simulink model "Simple_noL"  (R2020a)
settings: Solver=ode23  StartTime=0.0  StopTime=10.0  MaxStep=1e-2  RelTol=1e-3
libraries: simulink x4, fmu_me_lib x4
settings Model: Creator=Bob  LastModifiedBy=meagh
settings SFSimCC: CustomCodeUndefinedFunction=UseInterfaceOnly

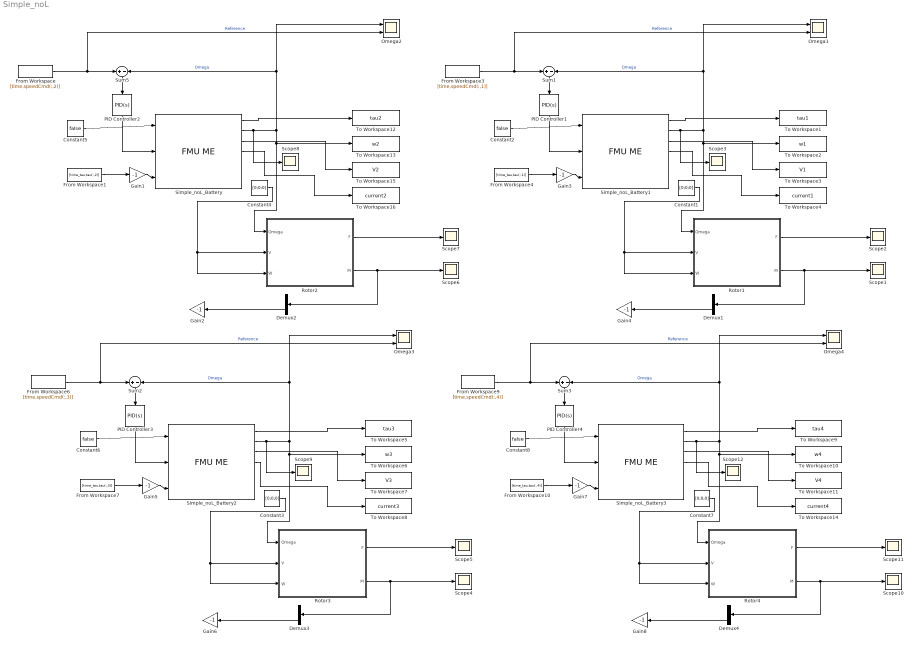
== system Simple_noL ==
  Constant{1,3..4,7} (4 alike) : Constant  Value=[0;0;0]
  Constant{2,5..6,8} (4 alike) : Constant  Value=false  OutDataTypeStr=boolean
  Demux{1..4} (4 alike) : Demux  Outputs=3
  From Workspace : FromWorkspace  VariableName=[time,speedCmd(:,2)]
  From Workspace1 : FromWorkspace  VariableName=[time_tau,tau(:,2)]
  From Workspace10 : FromWorkspace  VariableName=[time_tau,tau(:,4)]
  From Workspace3 : FromWorkspace  VariableName=[time,speedCmd(:,1)]
  From Workspace4 : FromWorkspace  VariableName=[time_tau,tau(:,1)]
  From Workspace6 : FromWorkspace  VariableName=[time,speedCmd(:,3)]
  From Workspace7 : FromWorkspace  VariableName=[time_tau,tau(:,3)]
  From Workspace9 : FromWorkspace  VariableName=[time,speedCmd(:,4)]
  Gain{1..8} (8 alike) : Gain  Gain=-1
  Omega{1..4} (4 alike) : Scope  NumInputPorts=2
  PID Controller{1..4} (4 alike) : simulink/Continuous/PID Controller  Controller=PID  Form=Parallel  TimeDomain=Continuous-time  UseExternalTs=off  SampleTime=-1  IntegratorMethod=Forward Euler  FilterMethod=Forward Euler  ControllerParametersSource=internal  P=0.0184*0.2  I=0.0184  D=0  UseFilter=on  N=100  TunerSelectOption=Transfer Function Based (PID Tuner App)  InitialConditionSource=internal  InitialConditionForIntegrator=0  InitialConditionForFilter=0  DifferentiatorICPrevScaledInput=0  ExternalReset=none  TrackingMode=off  Kt=1  LimitOutput=off  UpperSaturationLimit=inf  LowerSaturationLimit=-inf  LinearizeAsGain=on  AntiWindupMode=none  Kb=1  POutMin=[]  POutMax=[]  IOutMin=[]  IOutMax=[]  DOutMin=[]  DOutMax=[]  NOutMin=[]  NOutMax=[]  SumOutMin=[]  SumOutMax=[]  SaturationOutMin=[]  SaturationOutMax=[]  PParamMin=[]  PParamMax=[]  IParamMin=[]  IParamMax=[]  DParamMin=[]  DParamMax=[]  NParamMin=[]  NParamMax=[]  KbParamMin=[]  KbParamMax=[]  KtParamMin=[]  KtParamMax=[]  KbOutMin=[]  KbOutMax=[]  KtOutMin=[]  KtOutMax=[]  IntegratorOutMin=[]  IntegratorOutMax=[]  FilterOutMin=[]  FilterOutMax=[]  SumI1OutMin=[]  SumI1OutMax=[]  SumI2OutMin=[]  SumI2OutMax=[]  SumI3OutMin=[]  SumI3OutMax=[]  SumI4OutMin=[]  SumI4OutMax=[]  SumDOutMin=[]  SumDOutMax=[]  DifferentiatorOutMin=[]  DifferentiatorOutMax=[]  FilterDiffOutCoefMin=[]  FilterDiffOutCoefMax=[]  ReciprocalOutMin=[]  ReciprocalOutMax=[]  SumDenOutMin=[]  SumDenOutMax=[]  SumNumOutMin=[]  SumNumOutMax=[]  DivideOutMin=[]  DivideOutMax=[]  UdiffTsProdOutMin=[]  UdiffTsProdOutMax=[]  NTsProdOutMin=[]  NTsProdOutMax=[]  UintegralTsProdOutMin=[]  UintegralTsProdOutMax=[]  UngainTsProdOutMin=[]  UngainTsProdOutMax=[]  IntegratorContinuousStateAttributes=''  IntegratorStateMustResolveToSignalObject=off  IntegratorRTWStateStorageClass=Auto  FilterContinuousStateAttributes=''  FilterStateMustResolveToSignalObject=off  FilterRTWStateStorageClass=Auto  ParallelPVariant=InternalParameters  IdealPVariant=Disabled  IVariant=InternalParameters  DVariant=InternalParameters  IntegratorVariant=Continuous  SatVariant=Disabled  AWVariant=Passthrough  PCopyVariant=Disabled  TRVariant=Disabled  FdbkBlocksVariant=Forward  IdealPFdbkVariant=Disabled  SatFdbkVariant=Disabled  DerivativeFilterVariant=ContFilter  NVariant=InternalParameters  NCopyVariant=Disabled  FilterICVariant=InternalICsFilter  IntegratorICVariant=InternalICs  ExternalResetVariant=Disabled  TRSumVariant=Passthrough  SumFdbkVariant=Disabled  SumVariant=Sum_PID  TsampFilterVariant=InternalTs  TsampNgainVariant=Passthrough  TsampIntegralVariant=Passthrough
  Rotor1 : Subsystem
  Rotor2 : Subsystem
  Rotor3 : Subsystem
  Rotor4 : Subsystem
  Scope{1..12} (12 alike) : Scope
  Simple_noL_Battery{,1..3} (4 alike) : fmu_me_lib/FMU ME  Description=Simulates an FMU for Model Exchange 1.0 or Model Exchange 2.0.  dummy=0
  Sum{1..3,5} (4 alike) : Sum  Inputs=+|-
  To Workspace1 : ToWorkspace  VariableName=tau1  SaveFormat=Timeseries  SampleTime=-1
  To Workspace10 : ToWorkspace  VariableName=w4  SaveFormat=Timeseries  SampleTime=-1
  To Workspace11 : ToWorkspace  VariableName=V4  SaveFormat=Timeseries  SampleTime=-1
  To Workspace12 : ToWorkspace  VariableName=tau2  SaveFormat=Timeseries  SampleTime=-1
  To Workspace13 : ToWorkspace  VariableName=w2  SaveFormat=Timeseries  SampleTime=-1
  To Workspace14 : ToWorkspace  VariableName=current4  SaveFormat=Timeseries  SampleTime=-1
  To Workspace15 : ToWorkspace  VariableName=V2  SaveFormat=Timeseries  SampleTime=-1
  To Workspace16 : ToWorkspace  VariableName=current2  SaveFormat=Timeseries  SampleTime=-1
  To Workspace2 : ToWorkspace  VariableName=w1  SaveFormat=Timeseries  SampleTime=-1
  To Workspace3 : ToWorkspace  VariableName=V1  SaveFormat=Timeseries  SampleTime=-1
  To Workspace4 : ToWorkspace  VariableName=current1  SaveFormat=Timeseries  SampleTime=-1
  To Workspace5 : ToWorkspace  VariableName=tau3  SaveFormat=Timeseries  SampleTime=-1
  To Workspace6 : ToWorkspace  VariableName=w3  SaveFormat=Timeseries  SampleTime=-1
  To Workspace7 : ToWorkspace  VariableName=V3  SaveFormat=Timeseries  SampleTime=-1
  To Workspace8 : ToWorkspace  VariableName=current3  SaveFormat=Timeseries  SampleTime=-1
  To Workspace9 : ToWorkspace  VariableName=tau4  SaveFormat=Timeseries  SampleTime=-1
  wires:
  Constant5/1 -> Simple_noL_Battery/1
  Rotor2/1(F) -> Scope7/1
  Simple_noL_Battery/1 -> To Workspace12/1
  Simple_noL_Battery/4 -> To Workspace16/1
  Simple_noL_Battery/3 -> To Workspace15/1
  Simple_noL_Battery/2 -> Scope8/1, To Workspace13/1, Rotor2/1(Omega), Omega2/1, Sum5/2  "Omega"
  Rotor2/2(M) -> Demux2/1, Scope6/1
  Constant4/1 -> Rotor2/3(W), Rotor2/2(V)
  From Workspace/1 -> Omega2/2, Sum5/1  "Reference"
  Demux2/3 -> Gain2/1
  PID Controller2/1 -> Simple_noL_Battery/2
  Sum5/1 -> PID Controller2/1
  From Workspace1/1 -> Gain1/1
  Gain1/1 -> Simple_noL_Battery/3
  From Workspace3/1 -> Omega1/2, Sum1/1  "Reference"
  Gain3/1 -> Simple_noL_Battery1/3
  Simple_noL_Battery1/2 -> Scope3/1, To Workspace2/1, Rotor1/1(Omega), Omega1/1, Sum1/2  "Omega"
  Simple_noL_Battery1/3 -> To Workspace3/1
  PID Controller1/1 -> Simple_noL_Battery1/2
  Simple_noL_Battery1/1 -> To Workspace1/1
  Constant1/1 -> Rotor1/3(W), Rotor1/2(V)
  Rotor1/1(F) -> Scope2/1
  Demux1/3 -> Gain4/1
  Sum1/1 -> PID Controller1/1
  Constant2/1 -> Simple_noL_Battery1/1
  Rotor1/2(M) -> Demux1/1, Scope1/1
  Simple_noL_Battery1/4 -> To Workspace4/1
  From Workspace4/1 -> Gain3/1
  PID Controller3/1 -> Simple_noL_Battery2/2
  Simple_noL_Battery2/2 -> Scope9/1, To Workspace6/1, Rotor3/1(Omega), Omega3/1, Sum2/2  "Omega"
  Gain5/1 -> Simple_noL_Battery2/3
  From Workspace6/1 -> Omega3/2, Sum2/1  "Reference"
  From Workspace7/1 -> Gain5/1
  Simple_noL_Battery2/4 -> To Workspace8/1
  Sum2/1 -> PID Controller3/1
  Demux3/3 -> Gain6/1
  Constant3/1 -> Rotor3/3(W), Rotor3/2(V)
  Simple_noL_Battery2/3 -> To Workspace7/1
  Simple_noL_Battery2/1 -> To Workspace5/1
  Rotor3/2(M) -> Demux3/1, Scope4/1
  Rotor3/1(F) -> Scope5/1
  Constant6/1 -> Simple_noL_Battery2/1
  PID Controller4/1 -> Simple_noL_Battery3/2
  Simple_noL_Battery3/2 -> Scope12/1, To Workspace10/1, Rotor4/1(Omega), Omega4/1, Sum3/2  "Omega"
  Gain7/1 -> Simple_noL_Battery3/3
  From Workspace9/1 -> Omega4/2, Sum3/1  "Reference"
  From Workspace10/1 -> Gain7/1
  Simple_noL_Battery3/4 -> To Workspace14/1
  Sum3/1 -> PID Controller4/1
  Demux4/3 -> Gain8/1
  Constant7/1 -> Rotor4/3(W), Rotor4/2(V)
  Simple_noL_Battery3/3 -> To Workspace11/1
  Simple_noL_Battery3/1 -> To Workspace9/1
  Rotor4/2(M) -> Demux4/1, Scope10/1
  Rotor4/1(F) -> Scope11/1
  Constant8/1 -> Simple_noL_Battery3/1

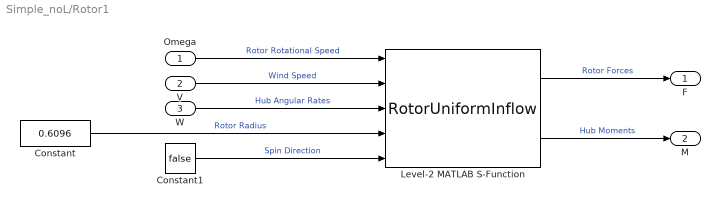
== system Simple_noL/Rotor1 ==
  Omega : Inport  OutDataTypeStr=double
  V : Inport  Port=2  OutDataTypeStr=double
  W : Inport  Port=3  OutDataTypeStr=double
  Constant : Constant  Value=0.6096
  Constant1 : Constant  Value=false  OutDataTypeStr=boolean
  Level-2 MATLAB S-Function : M-S-Function  FunctionName=RotorUniformInflow
  F : Outport  OutDataTypeStr=double  VectorParamsAs1DForOutWhenUnconnected=off
  M : Outport  Port=2  OutDataTypeStr=double  VectorParamsAs1DForOutWhenUnconnected=off
  wires:
  Level-2 MATLAB S-Function/2 -> M/1  "Hub Moments"
  Constant/1 -> Level-2 MATLAB S-Function/4  "Rotor Radius"
  Constant1/1 -> Level-2 MATLAB S-Function/5  "Spin Direction"
  Omega/1 -> Level-2 MATLAB S-Function/1  "Rotor Rotational Speed"
  V/1 -> Level-2 MATLAB S-Function/2  "Wind Speed"
  Level-2 MATLAB S-Function/1 -> F/1  "Rotor Forces"
  W/1 -> Level-2 MATLAB S-Function/3  "Hub Angular Rates"

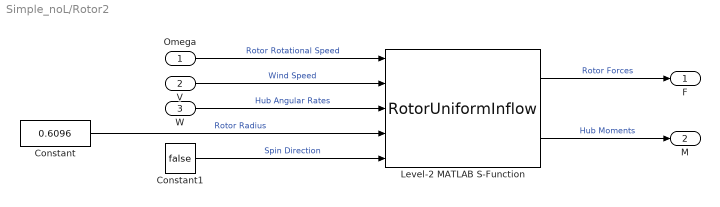
== system Simple_noL/Rotor2 ==
  Omega : Inport  OutDataTypeStr=double
  V : Inport  Port=2  OutDataTypeStr=double
  W : Inport  Port=3  OutDataTypeStr=double
  Constant : Constant  Value=0.6096
  Constant1 : Constant  Value=false  OutDataTypeStr=boolean
  Level-2 MATLAB S-Function : M-S-Function  FunctionName=RotorUniformInflow
  F : Outport  OutDataTypeStr=double  VectorParamsAs1DForOutWhenUnconnected=off
  M : Outport  Port=2  OutDataTypeStr=double  VectorParamsAs1DForOutWhenUnconnected=off
  wires:
  Level-2 MATLAB S-Function/2 -> M/1  "Hub Moments"
  Constant/1 -> Level-2 MATLAB S-Function/4  "Rotor Radius"
  Constant1/1 -> Level-2 MATLAB S-Function/5  "Spin Direction"
  Omega/1 -> Level-2 MATLAB S-Function/1  "Rotor Rotational Speed"
  V/1 -> Level-2 MATLAB S-Function/2  "Wind Speed"
  Level-2 MATLAB S-Function/1 -> F/1  "Rotor Forces"
  W/1 -> Level-2 MATLAB S-Function/3  "Hub Angular Rates"

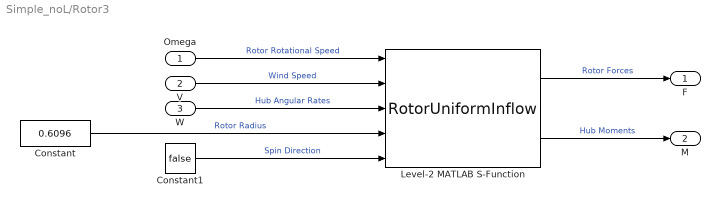
== system Simple_noL/Rotor3 ==
  Omega : Inport  OutDataTypeStr=double
  V : Inport  Port=2  OutDataTypeStr=double
  W : Inport  Port=3  OutDataTypeStr=double
  Constant : Constant  Value=0.6096
  Constant1 : Constant  Value=false  OutDataTypeStr=boolean
  Level-2 MATLAB S-Function : M-S-Function  FunctionName=RotorUniformInflow
  F : Outport  OutDataTypeStr=double  VectorParamsAs1DForOutWhenUnconnected=off
  M : Outport  Port=2  OutDataTypeStr=double  VectorParamsAs1DForOutWhenUnconnected=off
  wires:
  Level-2 MATLAB S-Function/2 -> M/1  "Hub Moments"
  Constant/1 -> Level-2 MATLAB S-Function/4  "Rotor Radius"
  Constant1/1 -> Level-2 MATLAB S-Function/5  "Spin Direction"
  Omega/1 -> Level-2 MATLAB S-Function/1  "Rotor Rotational Speed"
  V/1 -> Level-2 MATLAB S-Function/2  "Wind Speed"
  Level-2 MATLAB S-Function/1 -> F/1  "Rotor Forces"
  W/1 -> Level-2 MATLAB S-Function/3  "Hub Angular Rates"

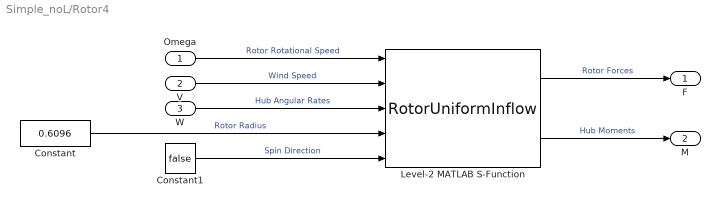
== system Simple_noL/Rotor4 ==
  Omega : Inport  OutDataTypeStr=double
  V : Inport  Port=2  OutDataTypeStr=double
  W : Inport  Port=3  OutDataTypeStr=double
  Constant : Constant  Value=0.6096
  Constant1 : Constant  Value=false  OutDataTypeStr=boolean
  Level-2 MATLAB S-Function : M-S-Function  FunctionName=RotorUniformInflow
  F : Outport  OutDataTypeStr=double  VectorParamsAs1DForOutWhenUnconnected=off
  M : Outport  Port=2  OutDataTypeStr=double  VectorParamsAs1DForOutWhenUnconnected=off
  wires:
  Level-2 MATLAB S-Function/2 -> M/1  "Hub Moments"
  Constant/1 -> Level-2 MATLAB S-Function/4  "Rotor Radius"
  Constant1/1 -> Level-2 MATLAB S-Function/5  "Spin Direction"
  Omega/1 -> Level-2 MATLAB S-Function/1  "Rotor Rotational Speed"
  V/1 -> Level-2 MATLAB S-Function/2  "Wind Speed"
  Level-2 MATLAB S-Function/1 -> F/1  "Rotor Forces"
  W/1 -> Level-2 MATLAB S-Function/3  "Hub Angular Rates"
